simulink model "mpc_ttype_psm"  (R2025b)
settings: Solver=ode23tb  StartTime=0.0  StopTime=simlength  FixedStep=tc  MaxStep=tc
values from neighbouring files (symbols this model uses):
  dead_time_INV = 1e-6    (= 1e-06)    [init_model.m]
  emf_fb_p = 0.2    [init_model.m]
  emf_fb_p_ccaller_1 = emf_fb_p    (= 0.2)    [init_model.m]
  emf_fb_p_ccaller_2 = emf_fb_p    (= 0.2)    [init_model.m]
  emf_p = emf_fb_p*4/10    (= 0.08)    [init_model.m]
  emf_p_ccaller_1 = emf_fb_p_ccaller_1*4/10    (= 0.08)    [init_model.m]
  emf_p_ccaller_2 = emf_fb_p_ccaller_2*4/10    (= 0.08)    [init_model.m]
  filters = setup_global_filters(ts_afe, ts_inv, ts_dab, tc)    [init_model.m]
  fPWM_INV = 6*fPWM    (= 24000)    [init_model.m]
  inv_m_scale = motorc_m_scale    [init_model.m]
  iq_lim = 1.4    [init_model.m]
  k_kalman = 0    [init_model.m]
  kg = Kobs(1)    [init_model.m]
  ki_w = 18    [init_model.m]
  kp_w = 2.5    [init_model.m]
  kw = Kobs(2)    [init_model.m]
  lim_down_align = -0.2    [init_model.m]
  lim_up_align = 0.2    [init_model.m]
  motorc_m_scale = 2/3*hwdata.inv.udc_nom/ubez    [init_model.m]
  number_of_modules = 1    [init_model.m]
  omega_m_sim = omega_m_bez    [init_model.m]
  simlength = 1.25    [init_model.m]
  tc = min(ts_afe)/400    [init_model.m]
  time_gain_afe_module_1 = 1.0    (= 1)    [init_model.m]
  time_gain_inv_module_1 = 1.0    (= 1)    [init_model.m]
  time_start_motor_control = 0.25    [init_model.m]
  torque_overload_factor = 1    [init_model.m]
  ts_inv = tPWM_INV    (= 4.16666666667e-05)    [init_model.m]
undefined symbols (not defined in the file or in its folder): A1_tilde_ekf, A2_tilde_ekf, A3_tilde_ekf, A4_tilde_ekf, Bd_ekf, C_ekf, hwdata, ibez, k_dc, k_sw, La, Lalpha_norm, Lb, Lbeta_norm, Ls_norm, omega_bez, omega_m_bez, psi_bez, psi_m, psi_m_norm, Qkalman, Rkalman, rpm_base, rpm_bez, Rs, Rs_norm, tau_bez, torque_base, ubez
libraries: fl_lib x25, nesl_utility x12, cstblocks x6, discrete_time_low_pass_filter x2, litium_ion_battery x1, dclink_for_three_levels x1, three_phase_three_level_ttype_inverter_ideal_switch_based_model x1, single_phase_pwm_modulator x1, threephase_inductor_lib x1, flexshaft_lib x1, psm x1
(part 4 of 4)

== matlab function mpc_ttype_psm/inv_psm_mod1/inverter_ctrl/inverter_control/inner_ctrl/mp control/mpc_pu_d ==
  data: S1a output; S2a output; S3a output; S4a output; S1b output; S2b output; S3b output; S4b output; S1c output; S2c output; S3c output; S4c output; vdc1 input; vdc2 input; ialpha_ref input; ibeta_ref input; ialpha input; ualpha output; ibeta input; omega_hat input; psi_alpha_hat input; psi_beta_hat input; ubeta output; Rs_norm parameter; Lalpha_norm parameter; Lbeta_norm parameter; ts_inv parameter; k_kalman parameter; omega_bez parameter; k_dc parameter; k_sw parameter
function [S1a, S2a, S3a, S4a, S1b, S2b, S3b, S4b, S1c, S2c, S3c, S4c, ualpha, ubeta] = mpc_ttype_gate(...
    vdc1, vdc2, ialpha_ref, ibeta_ref, ialpha, ibeta, ...
    omega_hat, psi_alpha_hat, psi_beta_hat, Rs_norm, Lalpha_norm, Lbeta_norm, ...
    ts_inv, k_kalman, omega_bez, k_dc, k_sw)
    
    % vdc1, vdc2: tensioni dei due condensatori (superiore e inferiore)
    % k_dc: peso per il bilanciamento del punto neutro nella funzione di costo
    
    persistent ualpha_prev ubeta_prev states_table
    
    if isempty(ualpha_prev)
        ualpha_prev = 0.0;
        ubeta_prev = 0.0;
        % Tabella dei 27 stati di commutazione [-1, 0, 1]
        states_table = [
            -1,-1,-1; -1,-1, 0; -1,-1, 1; -1, 0,-1; -1, 0, 0; -1, 0, 1; -1, 1,-1; -1, 1, 0; -1, 1, 1;
             0,-1,-1;  0,-1, 0;  0,-1, 1;  0, 0,-1;  0, 0, 0;  0, 0, 1;  0, 1,-1;  0, 1, 0;  0, 1, 1;
             1,-1,-1;  1,-1, 0;  1,-1, 1;  1, 0,-1;  1, 0, 0;  1, 0, 1;  1, 1,-1;  1, 1, 0;  1, 1, 1
        ];
    end

    Vdd = 15;
    ts = ts_inv * omega_bez;
    vdc_tot = vdc1 + vdc2;
    Vdc3 = vdc_tot / 3.0; 
    sqrt3_2 = 0.866025403784439;
    
    % Trasformazione inversa di Clarke per ottenere le correnti di fase attuali
    % Necessarie per calcolare la corrente del punto neutro i_np
    ia = ialpha;
    ib = -0.5 * ialpha + sqrt3_2 * ibeta;
    ic = -0.5 * ialpha - sqrt3_2 * ibeta;

    minJ = 1e18; 
    best_idx = 14; 
    ualpha = 0.0;
    ubeta = 0.0;

    for n = 1:27
        % 1. Tensioni candidate
        sa = states_table(n,1);
        sb = states_table(n,2);
        sc = states_table(n,3);
        
        ua = Vdc3 * (sa - 0.5*sb - 0.5*sc);
        ub = Vdc3 * (sqrt3_2 * sb - sqrt3_2 * sc);

        % 2. Predizione correnti
        ia_p = (1.0 - Rs_norm/Lalpha_norm*ts)*ialpha + (omega_hat/Lalpha_norm*psi_beta_hat*ts) + (ua*ts/Lalpha_norm);
        ib_p = (1.0 - Rs_norm/Lbeta_norm*ts)*ibeta - (omega_hat/Lbeta_norm*psi_alpha_hat*ts) + (ub*ts/Lbeta_norm);

        % 3. Bilanciamento Punto Neutro
        % La corrente che esce dal punto neutro (np) è data dalle fasi che sono nello stato '0'
        % i_np = (sa==0)*ia + (sb==0)*ib + (sc==0)*ic
        inp = double(sa==0)*ia + double(sb==0)*ib + double(sc==0)*ic;
        
        % Predizione dello sbilanciamento futuro (delta_v = vdc1 - vdc2)
        % Se inp > 0, il punto neutro si scarica, influenzando la differenza tra i condensatori
        % Assumendo C1 = C2 = C, la variazione della differenza di tensione è proporzionale a inp
        dv_future = (vdc1 - vdc2) + (1/1e-3) * inp * ts; % 1e-3 è una capacità fittizia, k_dc compenserà

        % 4. Funzione di Costo
        J_error = (ialpha_ref - ia_p)^2 + (ibeta_ref - ib_p)^2;
        J_sw = k_sw * ((ua - ualpha_prev)^2 + (ub - ubeta_prev)^2);
        J_dc = k_dc * (dv_future^2); % Termine di bilanciamento
        
        current_J = J_error + J_sw + J_dc;

        if current_J < minJ
            minJ = current_J;
            best_idx = n;
            ualpha = ua;
            ubeta = ub;
        end
    end

    ualpha_prev = ualpha;
    ubeta_prev = ubeta;

    % Decodifica Gate (identica a prima)
    ga = states_table(best_idx, 1);
    gb = states_table(best_idx, 2);
    gc = states_table(best_idx, 3);

    S1a = Vdd * double(ga == 1); S2a = Vdd * double(ga >= 0); S3a = Vdd * double(ga <= 0); S4a = Vdd * double(ga == -1);
    S1b = Vdd * double(gb == 1); S2b = Vdd * double(gb >= 0); S3b = Vdd * double(gb <= 0); S4b = Vdd * double(gb == -1);
    S1c = Vdd * double(gc == 1); S2c = Vdd * double(gc >= 0); S3c = Vdd * double(gc <= 0); S4c = Vdd * double(gc == -1);
end
